simulink model "pwmCnv"  (R2023b)
settings: Solver=FixedStepDiscrete  StartTime=0.0  StopTime=10.0  FixedStep=Ts  RelTol=1e-3  EnableMultiTasking=on
undefined symbols (not defined in the file): Ts
settings Model: RequirementInfo={} %GIDa_9cd6bfe3_9e51_41b9_91c5_89e7b64823b3  Creator=jrivitus  LastModifiedBy=student
settings SolverCC: MaxConsecutiveZCs=25  AlgebraicLoopSolver=TrustRegion
settings DataIOCC: DSMLogging=off  ReturnWorkspaceOutputs=off
settings OptimizationCC: DefaultParameterBehavior=Inlined  ExpressionDepthLimit=2147483647  InitFltsAndDblsToZero=on  LifeSpan=1  EfficientTunableParamExpr=on
settings DebuggingCC: UnderspecifiedInitializationDetection=Classic  MergeDetectMultiDrivingBlocksExec=none  ParameterPrecisionLossMsg=none  FcnCallInpInsideContextMsg=warning  UnconnectedInputMsg=warning  UnconnectedOutputMsg=warning  UnconnectedLineMsg=warning  AllowSymbolicDim=off  StateNameClashWarn=warning  PregeneratedLibrarySubsystemCodeDiagnostic=none  SFUnexpectedBacktrackingDiag=warning  SFNoUnconditionalDefaultTransitionDiag=warning  SFExecutionAtInitializationDiag=none  ArithmeticOperatorsInVariantConditions=warning
settings HardwareCC: ProdLongLongMode=on
settings ModelReferenceCC: UpdateModelReferenceTargets=IfOutOfDate  EnableRefExpFcnMdlSchedulingChecks=on  PropagateSignalLabelsOutOfModel=off
settings SFSimCC: SimUseLocalCustomCode=off  MATLABDynamicMemAlloc=off
settings RTWCC: Description=Embedded Coder  SystemTargetFile=ert.tlc  TemplateMakefile=ert_default_tmf  RTWUseLocalCustomCode=off  DLArmComputeVersion=19.05
settings CodeAppCC: IgnoreCustomStorageClasses=off  StateflowObjectComments=on
settings ERTTargetCC: MultiwordLength=2048  GenerateSampleERTMain=on  InlinedParameterPlacement=NonHierarchical  ERTCustomFileTemplate=example_file_process.tlc  ConvertIfToSwitch=off  SuppressUnreachableDefaultCases=off
settings ConfigComp: CovEnable=on  CovScope=ReferencedModels  RecordCoverage=on  CovMetricSettings=dcmwe  CovHTMLOptions=-sRT=1 -sVT=0 -aTS=1 -bRG=1 -bTC=1 -hTR=0 -nFC=0 -nFD=1 -scm=1 -bcm=1 -xEv=0 -xEM=0  CovSaveCumulativeToWorkspaceVar=on  CovModelRefEnable=Off  CovExternalEMLEnable=off  CovSFcnEnable=off  DVTestSuiteOptimization=CombinedObjectives (Nonlinear Extended)  DVIgnoreExistTestSatisfied=off

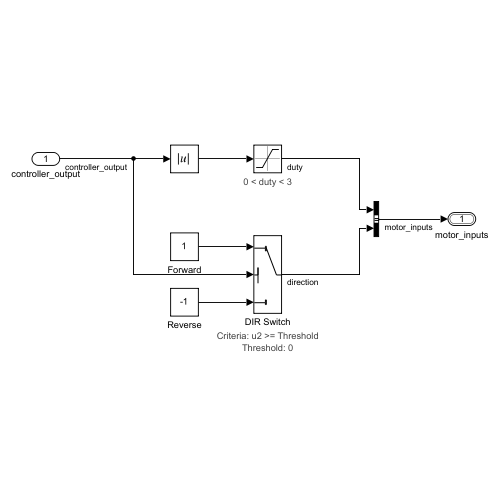
[thumbnail: Simulink's stored preview of the top-level diagram]
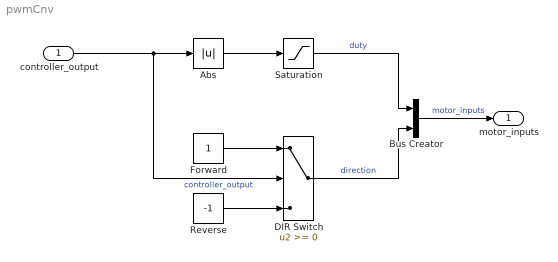
== system pwmCnv ==
  controller_output : Inport  OutDataTypeStr=double  PortDimensions=1  SampleTime=Ts
  Abs : Abs  SaturateOnIntegerOverflow=off
  Bus Creator : BusCreator  Inputs=2  OutDataTypeStr=Bus: motor_inputs_bus  NonVirtualBus=on
  DIR Switch : Switch  SaturateOnIntegerOverflow=off  InputSameDT=off
      settings: AttributesFormatString=Criteria: %<Criteria>\nThreshold: %<Threshold>
  Forward : Constant  OutDataTypeStr=double
  Reverse : Constant  Value=-1  OutDataTypeStr=double
  Saturation : Saturate  UpperLimit=3  LowerLimit=0
      settings: AttributesFormatString=%<LowerLimit> < duty < %<UpperLimit>
  motor_inputs : Outport  OutDataTypeStr=Bus: motor_inputs_bus  SampleTime=Ts  VectorParamsAs1DForOutWhenUnconnected=off  BusOutputAsStruct=on
  wires:
  Bus Creator/1 -> motor_inputs/1  "motor_inputs"
  Abs/1 -> Saturation/1
  Saturation/1 -> Bus Creator/1  "duty"
  DIR Switch/1 -> Bus Creator/2  "direction"
  Reverse/1 -> DIR Switch/3
  Forward/1 -> DIR Switch/1
  controller_output/1 -> DIR Switch/2, Abs/1  "controller_output"
